simulink model "analog_first_order_filter_with_step"  (R2020b)
settings: Solver=ode1be  StartTime=0.0  StopTime=30  RelTol=1e-3  AbsTol=1e-3
libraries: analogCompBlocks x8, fl_lib x3, nesl_utility x2
settings Model: DataDictionary=analogComputerData.sldd  EnableAccessToBaseWorkspace=off  OrderedModelArguments=off  Creator=roadrunner  LastModifiedBy=roadrunner
settings SolverCC: AutoScaleAbsTol=off
settings DebuggingCC: SymbolicDimsDataTypeCodeGenerationDiagnostic=none
settings SFSimCC: CustomCodeUndefinedFunction=UseInterfaceOnly
settings SimscapeCC: SimscapeLogType=all  SimscapeLogSimulationStatistics=on  SimscapeLogDataHistory=10000

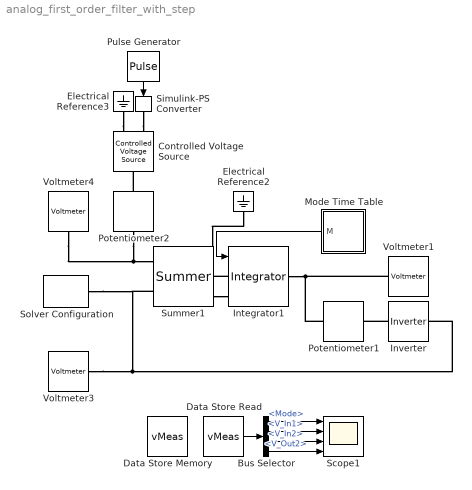
== system analog_first_order_filter_with_step ==
  Bus Selector : BusSelector  OutputSignals=Mode,V_In1,V_In2,V_Out2
  Controlled Voltage Source : fl_lib/Electrical/Electrical Sources/Controlled Voltage Source
      settings: AttributesFormatString=|
      | Input Step
      | Voltage
  Data Store Memory : DataStoreMemory  Priority=5  DataStoreName=vMeas  ReadBeforeWriteMsg=warning  WriteAfterWriteMsg=warning  WriteAfterReadMsg=warning  ShowAdditionalParam=off  OutDataTypeStr=Bus: bus_step_filter_measurements
  Data Store Read : DataStoreRead  Priority=6  DataStoreName=vMeas
  Electrical Reference2 : fl_lib/Electrical/Electrical Elements/Electrical Reference
  Electrical Reference3 : fl_lib/Electrical/Electrical Elements/Electrical Reference
  Integrator1 : analogCompBlocks/Integrator  capacitance=0.1  small_resistance=0.1  tau=0.1
      settings: AttributesFormatString=Integrator
  Inverter : analogCompBlocks/Inverter  SystemSampleTime=-1  VariantActivationTime=update diagram  Latency=0  AutoFrameSizeCalculation=off
      settings: AttributesFormatString=Inverter
  Mode Time Table : Subsystem  Priority=0  mask{DSNAME='vMeas', DSELEMENT='Mode'}
      mask prompts: DSNAME "Data Store Name"; DSELEMENT "Data Store Element"
      mask init:
      | % % Set data store name
      | % DSBLOCK = [gcb '/DataStoreWrite'];
      | % set_param(DSBLOCK,'DataStoreName',DSNAME)
      | % 
      | % % Set data store write element
      | % DSELEMENT = [DSNAME '.' DSELEMENT];
      | % set_param(DSBLOCK,'DataStoreElements',DSELEMENT)
      settings: AttributesFormatString=|
      | Mode Time
      | Table
  Potentiometer1 : analogCompBlocks/Potentiometer  wiper_position=10  max_resistance=1  gain=1
      settings: AttributesFormatString=|
      | Potentiometer
      | 1/tau
  Potentiometer2 : analogCompBlocks/Potentiometer  wiper_position=natural_frequency  max_resistance=1  gain=1
      settings: AttributesFormatString=|
      | Potentiometer
      | g/L
  Pulse Generator : DiscretePulseGenerator  PulseType=Time based  Period=20  PulseWidth=50  PhaseDelay=5
  Scope1 : Scope  NumInputPorts=4
  Simulink-PS Converter : nesl_utility/Simulink-PS Converter  PhysicalDomain=network_engine_domain  SubClassName=ps_input  LeftPortType=input  RightPortType=output  PseudoPeriodic=off  Frequencies=[]  NoiseDistribution=none  NoiseParameters=[]  Unit=V  AffineConversion=off  FilteringAndDerivatives=provide  SimscapeFilterOrder=1  InputFilterTimeConstant=0.001  UdotUserProvided=0
  Solver Configuration : nesl_utility/Solver Configuration  PhysicalDomain=network_engine_domain  SubClassName=solver  LeftPortType=input  RightPortType=generic  Tones=[]  Harmonics=[]  SimulateNoise=off  Profile=off  UseLocalSampling=off  EnableSwitchedLinearOptims=on  FrequencyDomain=off  UseCCode=off  RelTol=0.001  AbsTol=1e-06  MinStep=1e-09  ToWorkspace=off  RevertToSquareIcSolve=off  NumHomotopyIterations=100  PhasorMode=off  PhasorModeNumHarmonics=1  DoDC=off  ResidualTolerance=1e-09  UseLocalSolver=on  LocalSolverChoice=NE_BACKWARD_EULER_ADVANCER  LocalSolverSampleTime=0.001  DoFixedCost=on  MaxNonlinIter=3  MaxModeIter=2  ComputeImpulses=off  ImpulseIterations=2  LinearAlgebra=auto  EquationFormulation=NE_TIME_EF  DelaysMemoryBudget=1024  AutomaticFiltering=on  FilteringTimeConstant=0.001  PartitionStorageMethod=AS_NEEDED  PartitionMemoryBudget=1024  PartitionMethod=ROBUST
      settings: SourceProductName=Utilities
  Summer1 : analogCompBlocks/Summer  SystemSampleTime=-1  VariantActivationTime=update diagram  Latency=0  AutoFrameSizeCalculation=off
      settings: AttributesFormatString=Summer
  Voltmeter1 : analogCompBlocks/Voltmeter  Priority=4  DSNAME='vMeas'  DSELEMENT='V_Out2'
      settings: AttributesFormatString=|
      | Voltage Sensor
      | %<DSELEMENT>
  Voltmeter3 : analogCompBlocks/Voltmeter  Priority=4  DSNAME='vMeas'  DSELEMENT='V_In1'
      settings: AttributesFormatString=|
      | Voltage Sensor
      | %<DSELEMENT>
  Voltmeter4 : analogCompBlocks/Voltmeter  Priority=4  DSNAME='vMeas'  DSELEMENT='V_In2'
      settings: AttributesFormatString=|
      | Voltage Sensor
      | %<DSELEMENT>
  wires:
  Data Store Read/1 -> Bus Selector/1
  Mode Time Table/1(M) -> Integrator1/1
  Pulse Generator/1 -> Simulink-PS Converter/1
  Bus Selector/1 -> Scope1/1  "<Mode>"
  Bus Selector/2 -> Scope1/2  "<V_In1>"
  Bus Selector/3 -> Scope1/3  "<V_In2>"
  Bus Selector/4 -> Scope1/4  "<V_Out2>"
  connections:
  Integrator1/LConn1 -- Summer1/RConn1
  Potentiometer1/LConn1 -- Voltmeter1/LConn1 -- Integrator1/RConn1
  Electrical Reference2/LConn1 -- Integrator1/LConn2
  Inverter/LConn1 -- Potentiometer1/RConn1
  Voltmeter4/LConn1 -- Potentiometer2/RConn1 -- Summer1/LConn1
  Simulink-PS Converter/RConn1 -- Controlled Voltage Source/RConn1
  Electrical Reference3/LConn1 -- Controlled Voltage Source/RConn2
  Voltmeter3/LConn1 -- Inverter/RConn1 -- Solver Configuration/RConn1 -- Summer1/LConn2
  Potentiometer2/LConn1 -- Controlled Voltage Source/LConn1

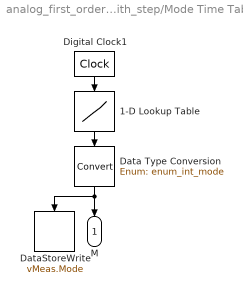
== system analog_first_order_filter_with_step/Mode Time Table ==
  1-D Lookup Table : Lookup_n-D  NumberOfTableDimensions=1  BreakpointsForDimension1=[0 1 28]  Table=[0 2 1]  InterpMethod=Flat  ExtrapMethod=Clip  InternalRulePriority=Speed  OutDataTypeStr=int32  RndMeth=Simplest  InputSameDT=on
      settings: AttributesFormatString=|
      | Integrator Mode
      | Time Table
  Data Type Conversion : DataTypeConversion  OutDataTypeStr=Enum: enum_int_mode
      settings: AttributesFormatString=|
      | Convert to
      | Mode Enum
  DataStoreWrite : DataStoreWrite  DataStoreName=vMeas  DataStoreElements=vMeas.Mode
  Digital Clock1 : DigitalClock  SampleTime=0.01
      settings: AttributesFormatString=Timer
  M : Outport
  wires:
  1-D Lookup Table/1 -> Data Type Conversion/1
  Digital Clock1/1 -> 1-D Lookup Table/1
  Data Type Conversion/1 -> DataStoreWrite/1, M/1
